simulink model "B2B_HVDC_MMC"  (R2023b)
settings: Solver=ode23t  StartTime=0.0  StopTime=3  FixedStep=Ts_Power  MaxStep=1e-3  MinStep=Ts_Power  RelTol=1e-3
values from neighbouring files (symbols this model uses):
  AC_lim = 1*[1.5 -1.5]    [B2B_HVDC_MMC_Calc.m]
  C_pm = 10.48e-3    (= 0.01048)    [B2B_HVDC_MMC_Calc.m]
  Carm = 1.0*C_pm/n    (= 0.0002096)    [B2B_HVDC_MMC_Calc.m]    (also in HVDC_MMC_param.m = 4.88333333333e-05)
  ccsc_lim = 1*[1.0 -1.0]    [B2B_HVDC_MMC_Calc.m]
  DC_lim = 1*[1.05 -1.05]    [B2B_HVDC_MMC_Calc.m]
  f = 50    [B2B_HVDC_MMC_Calc.m]
  Fn_filter = 1000    [B2B_HVDC_MMC_Calc.m]    (also in HVDC_MMC_param.m)
  Fnom = 50    [HVDC_MMC_param.m]
  HrmOrd = N    (= 2)    [B2B_HVDC_MMC_Calc.m]    (also in HVDC_MMC_param.m)
  I_nom = S_nom/(sqrt(3)*V_grid)    [B2B_HVDC_MMC_Calc.m]
  Ireg_lim_i = 1*[1.5, -1.5]    [B2B_HVDC_MMC_Calc.m]
  Ireg_lim_r = 2*[1.5, -1.5]    [B2B_HVDC_MMC_Calc.m]
  Ki_ACreg_i = 260    [B2B_HVDC_MMC_Calc.m]
  Ki_ccsc = 5    [B2B_HVDC_MMC_Calc.m]
  Ki_DCreg_r = 150    [B2B_HVDC_MMC_Calc.m]
  Ki_Ireg_i = 200    [B2B_HVDC_MMC_Calc.m]
  Ki_Ireg_r = 50    [B2B_HVDC_MMC_Calc.m]
  Kp_ACreg_i = 2    [B2B_HVDC_MMC_Calc.m]
  Kp_ccsc = 1    [B2B_HVDC_MMC_Calc.m]
  Kp_DCreg_r = 8    [B2B_HVDC_MMC_Calc.m]
  Kp_Ireg_i = 2    [B2B_HVDC_MMC_Calc.m]
  Kp_Ireg_r = 0.8    [B2B_HVDC_MMC_Calc.m]
  L1_si = L1_pu*Z_base66/w    [B2B_HVDC_MMC_Calc.m]
  L_arm = L_arm_pu*Z_base66/w    [B2B_HVDC_MMC_Calc.m]
  L_arm_pu = 0.15    [B2B_HVDC_MMC_Calc.m]
  N = 2    [B2B_HVDC_MMC_Calc.m]
  P_nom = 220e6    (= 220000000)    [B2B_HVDC_MMC_Calc.m]
  R1_si = R1_pu*Z_base66    [B2B_HVDC_MMC_Calc.m]
  R_arm = 0.03    [B2B_HVDC_MMC_Calc.m]
  R_arm_pu = R_arm/Z_base66    [B2B_HVDC_MMC_Calc.m]
  R_load = 0.6*40    (= 24)    [B2B_HVDC_MMC_Calc.m]
  R_startup = 17    [B2B_HVDC_MMC_Calc.m]    (also in HVDC_MMC_param.m = 400)
  T_fault = 1.4    [B2B_HVDC_MMC_Calc.m]
  Ts = Ts_Power    (= 5e-05)    [B2B_HVDC_MMC_Calc.m]    (also in HVDC_MMC_param.m)
  Ts_Control = Ts_Power    (= 5e-05)    [B2B_HVDC_MMC_Calc.m]    (also in HVDC_MMC_param.m)
  Ts_DQN = MultTs*Ts_Power    (= 5e-05)    [B2B_HVDC_MMC_Calc.m]    (also in HVDC_MMC_param.m)
  Ts_Power = 1*50e-6    (= 5e-05)    [B2B_HVDC_MMC_Calc.m]    (also in HVDC_MMC_param.m)
  V_ac_ref = 1.035    [B2B_HVDC_MMC_Calc.m]
  V_grid = 66e3    (= 66000)    [B2B_HVDC_MMC_Calc.m]
  Vdc_nom = 135e3    (= 135000)    [B2B_HVDC_MMC_Calc.m]
  Vnom_prim = 333e3    (= 333000)    [HVDC_MMC_param.m]
  Xdcpnz = [zeros(6,1), Xpnz]    [B2B_HVDC_MMC_Calc.m]
  Zeta_filter = 1    [B2B_HVDC_MMC_Calc.m]    (also in HVDC_MMC_param.m)
undefined symbols (not defined in the file or in its folder): DiscIntNeverNeededParam, Pcc, Xdcpnz_c
libraries: DQN_Lib x39, simulink x26, eeTransforms x21, spsCurrentMeasurementLib x16, spsHalfBridgeMMCLib x12, spsSeriesRLCBranchLib x12, B2B_HVDC_MMC_Lib x8, spsSecondOrderFilterLib x8, spsAlphaBetaZerotodq0Lib x6, spsabctoAlphaBetaZeroLib x6, spsThreePhaseVIMeasurementLib x4, spsabctodq0Lib x3
(part 2 of 5)

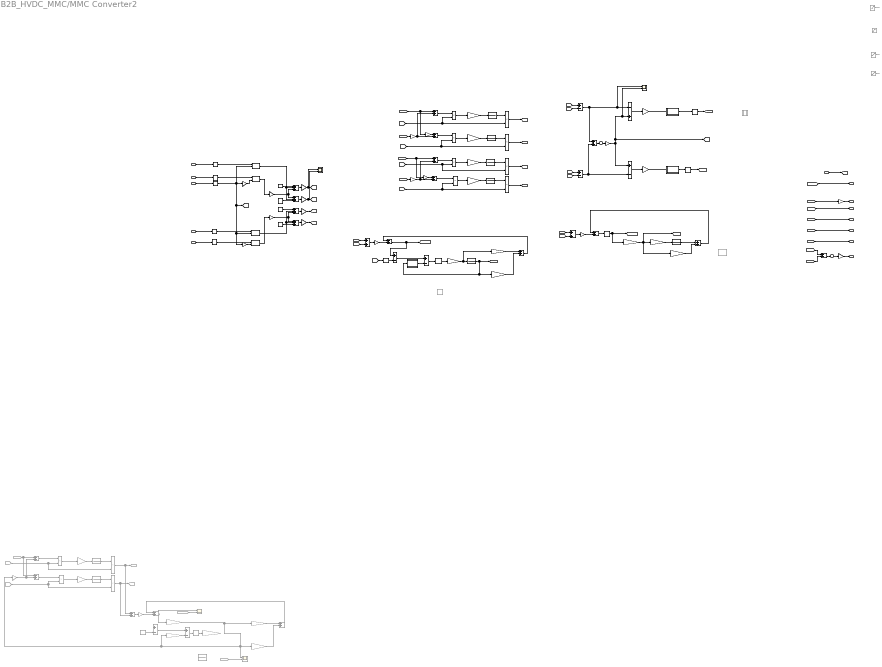
== system B2B_HVDC_MMC/MMC Converter2 ==
  m_dq1_r : Inport
  m_dq2_r : Inport  Port=2
  Vg : Inport  Port=3
  wt : Inport  Port=4
  m_dq1_i : Inport  Port=5
  m_dq2_i : Inport  Port=6
  Add1 : Sum  Inputs=+-
  Add{3,6,38..39,41,44,48,50,73} (9 alike) : Sum
  Add35 : Sum  Commented=on
  Add36 : Sum  Commented=on
  Add37 : Sum  Commented=on  Inputs=-+
  Add4 : Sum  Commented=on
  Add42 : Sum  Inputs=-+
  Add45 : Sum  Inputs=-+
  Add46 : Sum  Inputs=+-
  Add47 : Sum  Inputs=+-
  Add5 : Sum  Commented=on  Inputs=-+
  Constant : Constant  Commented=on  Value=0
  Constant{1..2,74..75} (4 alike) : Constant
  Delay : Delay  Commented=on  DelayLength=1  SampleTime=Ts_Power
  Delay{2..3,8..9} (4 alike) : Delay  DelayLength=1  SampleTime=Ts_Power
  Delay4 : Delay  Commented=on  DelayLength=1  SampleTime=Ts_Power
  Discrete Derivative : simulink/Discrete/Discrete Derivative  Commented=on  gainval=Ts_Power  ICPrevScaledInput=0.0  OutMin=[]  OutMax=[]  OutDataType=fixdt(1, 16)  OutScaling=2^-10  DoSatur=off
  Discrete-Time Integrator{,2..3,7,10..11} (6 alike) : DiscreteIntegrator  IntegratorMethod=Integration: Trapezoidal  SampleTime=Ts_Power  ICPrevOutput=DiscIntNeverNeededParam  ICPrevScaledInput=DiscIntNeverNeededParam
  Discrete-Time Integrator4 : DiscreteIntegrator  Commented=on  IntegratorMethod=Integration: Trapezoidal  SampleTime=Ts_Power  ICPrevOutput=DiscIntNeverNeededParam  ICPrevScaledInput=DiscIntNeverNeededParam
  Discrete-Time Integrator5 : DiscreteIntegrator  Commented=on  IntegratorMethod=Integration: Trapezoidal  SampleTime=Ts_Power  ICPrevOutput=DiscIntNeverNeededParam  ICPrevScaledInput=DiscIntNeverNeededParam
  Discrete-Time Integrator8 : DiscreteIntegrator  Commented=on  IntegratorMethod=Integration: Trapezoidal  SampleTime=Ts_Power  ICPrevOutput=DiscIntNeverNeededParam  ICPrevScaledInput=DiscIntNeverNeededParam
  From108 : From  Commented=on  GotoTag=Id_abc_i
  From51 : From  Commented=on  GotoTag=mn_i
  From56 : From  Commented=on  GotoTag=mp_i
  From72 : From  Commented=on  GotoTag=Ig_abc_i
  From75 : From  Commented=on  GotoTag=Vconv_i
  Gain{1..2,18,23..24} (5 alike) : Gain  Gain=-1
  Gain10 : Gain  Gain=1/6
  Gain12 : Gain  Gain=-2
  Gain13 : Gain  Commented=on  Gain=1/(Carm)
  Gain14 : Gain  Commented=on  Gain=1/(Carm)
  Gain15 : Gain  Commented=on  Gain=0.5
  Gain{4,21,39,43} (4 alike) : Gain  Gain=1/(Carm)
  Gain40 : Gain  Commented=on  Gain=-0.5
  Gain41 : Gain  Gain=1/2
  Gain44 : Gain  Gain=0.5
  Gain46 : Gain  Commented=on  Gain=1/R_load
  Gain47 : Gain  Gain=0.5
  Gain49 : Gain  Gain=-0.5
  Gain50 : Gain  Gain=1/R_load
  Gain51 : Gain  Gain=R_arm/2
  Gain52 : Gain  Commented=on  Gain=R_arm/2
  Gain53 : Gain  Commented=on  Gain=L_arm/2
  Gain54 : Gain  Commented=on  Gain=1/L1_si
  Gain55 : Gain  Commented=on  Gain=R1_si+R_load
  Gain56 : Gain  Gain=L_arm/2
  Gain60 : Gain  Gain=-0.5
  Gain61 : Gain  Gain=R_arm/2
  Gain62 : Gain  Gain=L_arm/2
  Gain65 : Gain  Gain=1/L1_si
  Gain9 : Gain  Gain=-2
  Goto56 : Goto  Commented=on  GotoTag=Vp_ic
  Goto57 : Goto  Commented=on  GotoTag=Vn_ic
  I->pu{1..3,5,22,28} (6 alike) : Gain  Gain=1/2  SaturateOnIntegerOverflow=on  OutDataTypeStr=Inherit: Same as input  ParamDataTypeStr=Inherit: Same as input
  Int : MATLAB Function  TreatAsAtomicUnit=on  mask{dt=Ts_Power}
      mask prompts: dt "Time step (s):"
  Int2 : MATLAB Function  TreatAsAtomicUnit=on  mask{dt=Ts_Power}
      mask prompts: dt "Time step (s):"
  Inverse Park Transform{1..4} (4 alike) : eeTransforms/Inverse Park Transform  AxisAlignment=Q-axis  PowerInvariant=off
  Product{1..3,5} (4 alike) : Product  Commented=on
  Product{4,6..12} (8 alike) : Product
  R_rec1 : Subsystem
  Rate Transition{1..4,10..11} (6 alike) : RateTransition  Integrity=off  OutPortSampleTimeMultiple=MultTs  OutPortSampleTime=Ts_Power
  Saturation3 : Saturate  Commented=on  UpperLimit=inf  LowerLimit=0  ZeroCross=off
  Saturation4 : Saturate  Commented=on  UpperLimit=inf  LowerLimit=0  ZeroCross=off
  Saturation5 : Saturate  Commented=on  UpperLimit=0  LowerLimit=-inf  ZeroCross=off
  Saturation6 : Saturate  Commented=on  UpperLimit=0  LowerLimit=-inf  ZeroCross=off
  Scope : Scope  NumInputPorts=2
  Scope1 : Scope  NumInputPorts=2
  Scope15 : Scope  Commented=on  NumInputPorts=2
  Scope8 : Scope  Commented=on  NumInputPorts=2
  Subsystem2 : Subsystem  Commented=on  mask{Ts_Power=Ts_Power, SW=off}
      mask prompts: Ts_Power "Sample time (s):"; SW "Fancy delay"
  Subtract1 : Sum  Inputs=+-+
  Subtract10 : Sum  Inputs=+-
  Subtract11 : Sum  Inputs=+-
  Subtract2 : Sum  Inputs=+-+
  Subtract3 : Sum  Inputs=+++
  Subtract4 : Sum  Commented=on  Inputs=+-
  Subtract5 : Sum  Inputs=+++
  Subtract8 : Sum  Commented=on  Inputs=+-
  Sum11 : Sum  Inputs=+-  InputSameDT=on  SaturateOnIntegerOverflow=on  OutDataTypeStr=Inherit: Same as first input
  Sum19 : Sum  Inputs=+
  Sum23 : Sum  Inputs=+
  Sum4 : Sum  Inputs=-+  InputSameDT=on  SaturateOnIntegerOverflow=on  OutDataTypeStr=Inherit: Same as first input
  Id_abc_i : Outport  VectorParamsAs1DForOutWhenUnconnected=off
  Ig_abc_i : Outport  Port=2  VectorParamsAs1DForOutWhenUnconnected=off
  Vg_abc_i : Outport  Port=3  VectorParamsAs1DForOutWhenUnconnected=off
  Idc : Outport  Port=4  VectorParamsAs1DForOutWhenUnconnected=off
  Ig_abc_r : Outport  Port=5  VectorParamsAs1DForOutWhenUnconnected=off
  Id_abc_r : Outport  Port=6  VectorParamsAs1DForOutWhenUnconnected=off
  Vdc : Outport  Port=7  VectorParamsAs1DForOutWhenUnconnected=off
  wires:
  Gain9/1 -> Inverse Park Transform2/2
  [mn_r] -> Product7/2, Product8/2
  Gain4/1 -> Discrete-Time Integrator3/1  "dVp_M"
  Gain21/1 -> Discrete-Time Integrator2/1  "dVn_M"
  Discrete-Time Integrator2/1 -> Product8/1  "Vn_M"
  Product4/1 -> Gain4/1
  Add6/1 -> Product7/1
  Add46/1 -> Scope1/1, Sum4/1, Add73/1  "dVp_M"
  Discrete-Time Integrator3/1 -> Product6/1  "Vp_M"
  Product7/1 -> Gain21/1
  Subtract2/1 -> I->pu22/1
  Constant74/1 -> Subtract2/1
  Inverse Park Transform2/1 -> Gain1/1
  Constant75/1 -> Subtract5/3
  Subtract5/1 -> I->pu28/1
  I->pu28/1 -> Scope/2, [mn_r]
  Inverse Park Transform1/1 -> Subtract5/2, Subtract2/2
  Gain12/1 -> Inverse Park Transform4/2
  wt/1 -> Rate Transition1/1
  Constant2/1 -> Subtract3/3
  Subtract1/1 -> I->pu2/1
  Constant1/1 -> Subtract1/1
  Subtract3/1 -> I->pu3/1
  I->pu2/1 -> [mp_i]
  Inverse Park Transform4/1 -> Gain2/1
  I->pu3/1 -> [mn_i]
  Gain15/1 -> Add4/2, Add5/2
  Discrete-Time Integrator5/1 -> Product2/1  "Vp_M"
  Add5/1 -> Product3/1
  Add4/1 -> Product1/1  "prod"
  Gain14/1 -> Discrete-Time Integrator5/1  "dVp_M"
  Product1/1 -> Gain14/1
  Discrete-Time Integrator4/1 -> Product5/1  "Vn_M"
  Gain13/1 -> Discrete-Time Integrator4/1  "dVn_M"
  Product3/1 -> Gain13/1
  From51/1 -> Product2/2, Product1/2
  From56/1 -> Product3/2, Product5/2
  Vg/1 -> [Vg_r]
  Sum4/1 -> I->pu5/1
  Gain23/1 -> Ig_abc_r/1
  Gain44/1 -> Add6/2, Add3/2
  From75/1 -> Scope8/2
  Constant/1 -> Subtract4/2
  Delay4/1 -> Gain54/1
  Gain55/1 -> Subtract8/2
  Subtract8/1 -> Delay4/1
  Gain53/1 -> Add36/1  "dVp_M"
  Gain52/1 -> Add36/2  "dVp_M"
  Add37/1 -> Scope8/1, Gain46/1  "prod"
  Subtract4/1 -> Subtract8/1
  Product2/1 -> Add35/1, Goto56/1
  Gain46/1 -> Scope15/1, Gain55/1, Gain15/1, Gain52/1, Gain53/1  "Igd"
  Product5/1 -> Add35/2, Goto57/1
  From72/1 -> Scope15/2
  Add36/1 -> Add37/1  "prod"
  Add35/1 -> Gain40/1
  Gain40/1 -> Add37/2  "Vce_i"
  From108/1 -> Add5/1, Add4/1
  Gain47/1 -> Add38/2, Add39/2
  Product11/1 -> Gain39/1
  [mp_i] -> Product11/2, Product12/2
  Add38/1 -> Product9/1  "prod"
  Discrete-Time Integrator11/1 -> Product10/1  "Vp_M"
  Gain39/1 -> Discrete-Time Integrator10/1  "dVn_M"
  Discrete-Time Integrator10/1 -> Product12/1  "Vn_M"
  Product9/1 -> Gain43/1
  Gain43/1 -> Discrete-Time Integrator11/1  "dVp_M"
  Add39/1 -> Product11/1
  [mn_i] -> Product10/2, Product9/2
  Add41/1 -> Add42/1  "prod"
  Gain51/1 -> Add41/2  "dVp_M"
  Add50/1 -> Gain49/1
  Gain49/1 -> Add42/2  "Vce_i"
  Subtract10/1 -> Subtract11/1
  Gain61/1 -> Add44/2  "dVp_M"
  Add44/1 -> Add45/1  "prod"
  Gain60/1 -> Add45/2  "Vce_r"
  Gain62/1 -> Add44/1  "dVp_M"
  R_rec1/1(Out) -> Subtract11/2
  Gain65/1 -> Discrete-Time Integrator/1, Gain62/1
  Add48/1 -> Gain60/1
  [Ig_abc_ic] -> Gain47/1
  [Id_abc_ic] -> Gain24/1, Add38/1
  [Vp_rc] -> Add46/1
  [Vn_rc] -> Add46/2
  [Vp_ic] -> Add47/1
  [Vn_ic] -> Add47/2
  [Ig_abc_rc] -> Gain44/1
  [Id_abc_rc] -> Add3/1, Gain18/1
  [Vp_rc] -> Add48/1
  [Vn_rc] -> Add48/2
  [Vp_ic] -> Add50/1
  [Vn_ic] -> Add50/2
  Add47/1 -> Sum11/2, Add73/2  "dVp_M"
  [Ig_abc_rc] -> Gain23/1
  [Id_abc_rc] -> Id_abc_r/1
  [Ig_abc_ic] -> Ig_abc_i/1
  [Id_abc_ic] -> Id_abc_i/1
  [Id_abc_rc] -> Add1/2
  Gain56/1 -> Discrete-Time Integrator7/1  "dVp_M"
  Discrete-Time Integrator7/1 -> Add41/1
  [Id_abc_ic] -> Add1/1
  Add1/1 -> Sum23/1
  Gain41/1 -> Idc/1  "Vce_r"
  Discrete-Time Integrator/1 -> [Ig_abc_rc], R_rec1/1(In), Gain61/1  "Igd"
  Add45/1 -> [Vconv_rc], Subtract10/1  "prod"
  Gain50/1 -> Gain51/1, [Ig_abc_ic], Gain56/1  "Igd"
  Add42/1 -> Delay8/1  "prod"
  [Vconv_ic] -> Vg_abc_i/1
  [V_dc_c] -> Vdc/1
  Subtract11/1 -> Delay9/1
  Gain1/1 -> Subtract5/1, Subtract2/3
  Inverse Park Transform3/1 -> Subtract1/2, Subtract3/2
  Gain2/1 -> Subtract3/1, Subtract1/3
  Gain10/1 -> Sum11/1, [V_dc_c], Scope1/2, Sum4/2  "Vce_r"
  m_dq2_r/1 -> Rate Transition11/1
  m_dq1_r/1 -> Rate Transition10/1
  m_dq1_i/1 -> Rate Transition2/1
  m_dq2_i/1 -> Rate Transition3/1
  Gain18/1 -> Add6/1
  Gain24/1 -> Add39/1
  Saturation4/1 -> ?
  Saturation3/1 -> ?
  Saturation6/1 -> ?
  Add73/1 -> Sum19/1
  Sum19/1 -> Gain10/1
  Int/1(z) -> Delay2/1
  Sum11/1 -> I->pu1/1
  Int2/1(z) -> Delay3/1
  Product6/1 -> [Vp_rc]
  Product8/1 -> [Vn_rc]
  Product10/1 -> [Vp_ic]
  Product12/1 -> [Vn_ic]
  Delay2/1 -> [Id_abc_rc]
  Delay3/1 -> [Id_abc_ic]
  Delay9/1 -> Gain65/1
  Delay8/1 -> Gain50/1, [Vconv_ic]
  I->pu5/1 -> Int/1(x)
  I->pu1/1 -> Int2/1(x)
  Rate Transition10/1 -> Inverse Park Transform1/1
  Rate Transition11/1 -> Inverse Park Transform2/1
  Rate Transition1/1 -> [wt], Inverse Park Transform3/2, Gain12/1, Inverse Park Transform1/2, Gain9/1
  Rate Transition2/1 -> Inverse Park Transform3/1
  Rate Transition3/1 -> Inverse Park Transform4/1
  [Vg_r] -> Rate Transition4/1
  Rate Transition4/1 -> Subtract10/2
  Sum23/1 -> Gain41/1
  I->pu22/1 -> Scope/1, [mp_r]
  Add3/1 -> Product4/1  "prod"
  [mp_r] -> Product4/2, Product6/2

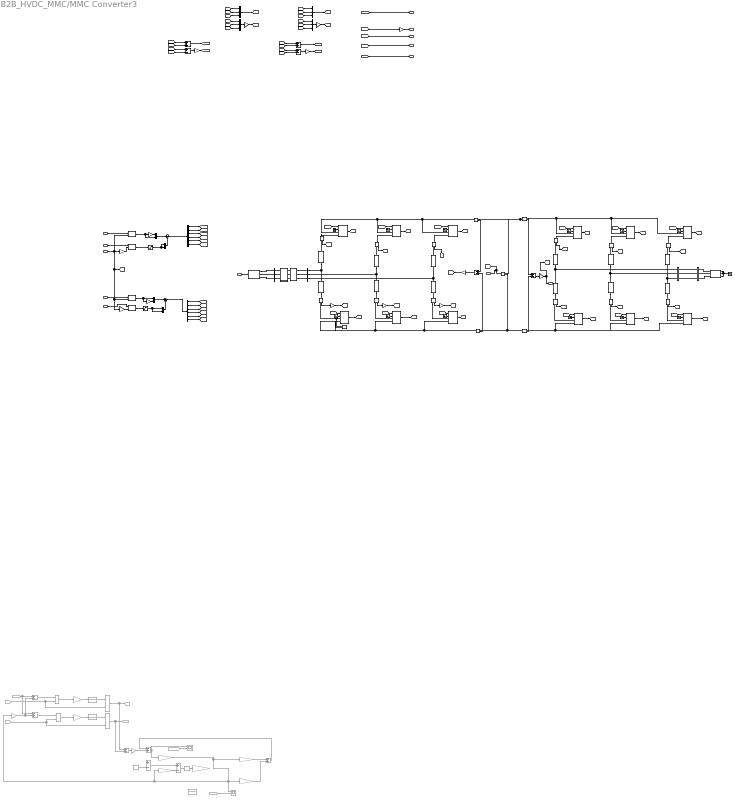
== system B2B_HVDC_MMC/MMC Converter3 ==
  m_dq1_r : Inport
  m_dq2_r : Inport  Port=2
  wt : Inport  Port=3
  V_Src : Inport  Port=4
  m_dq1_i : Inport  Port=5
  m_dq2_i : Inport  Port=6
  A1 : spsThreePhaseVIMeasurementLib/Three-Phase V-I Measurement  VoltageMeasurement=phase-to-ground  SetLabelV=on  LabelV=Vconv_r  Vpu=off  VpuLL=off  CurrentMeasurement=yes  SetLabelI=on  LabelI=Ig_r  Ipu=off  Pbase=100e6  Vbase=500e3  OutputType=Complex  PhasorSimulation=off  PSBequivalent=0
  A2 : spsThreePhaseVIMeasurementLib/Three-Phase V-I Measurement  VoltageMeasurement=phase-to-ground  SetLabelV=on  LabelV=Vconv_i  Vpu=off  VpuLL=off  CurrentMeasurement=yes  SetLabelI=on  LabelI=Ig_i  Ipu=off  Pbase=100e6  Vbase=500e3  OutputType=Complex  PhasorSimulation=off  PSBequivalent=0
  A3 : spsThreePhaseVIMeasurementLib/Three-Phase V-I Measurement  VoltageMeasurement=phase-to-ground  SetLabelV=on  LabelV=VA1  Vpu=off  VpuLL=off  CurrentMeasurement=yes  SetLabelI=on  LabelI=IA1  Ipu=off  Pbase=100e6  Vbase=500e3  OutputType=Complex  PhasorSimulation=off  PSBequivalent=0
  Add : Sum
  Add{8,11,13,51} (4 alike) : Sum  Inputs=+-
  Add35 : Sum  Commented=on
  Add36 : Sum  Commented=on
  Add37 : Sum  Commented=on  Inputs=-+
  Add4 : Sum  Commented=on
  Add40 : Sum
  Add5 : Sum  Commented=on  Inputs=-+
  B1 : spsThreePhaseVIMeasurementLib/Three-Phase V-I Measurement  VoltageMeasurement=phase-to-ground  SetLabelV=on  LabelV=VB1  Vpu=off  VpuLL=off  CurrentMeasurement=yes  SetLabelI=on  LabelI=IB1  Ipu=off  Pbase=100e6  Vbase=500e3  OutputType=Complex  PhasorSimulation=off  PSBequivalent=0
  Constant : Constant  Commented=on  Value=0
  Current Measurement{,1..15} (16 alike) : spsCurrentMeasurementLib/Current Measurement  PhasorSimulation=off  OutputType=Complex  PSBequivalent=0
  Delay4 : Delay  Commented=on  DelayLength=1  SampleTime=Ts_Power
  Demux1 : Demux  Outputs=6
  Demux2 : Demux  Outputs=6
  Discrete-Time Integrator4 : DiscreteIntegrator  Commented=on  IntegratorMethod=Integration: Trapezoidal  SampleTime=Ts_Power  ICPrevOutput=DiscIntNeverNeededParam  ICPrevScaledInput=DiscIntNeverNeededParam
  Discrete-Time Integrator5 : DiscreteIntegrator  Commented=on  IntegratorMethod=Integration: Trapezoidal  SampleTime=Ts_Power  ICPrevOutput=DiscIntNeverNeededParam  ICPrevScaledInput=DiscIntNeverNeededParam
  Discrete-Time Integrator8 : DiscreteIntegrator  Commented=on  IntegratorMethod=Integration: Trapezoidal  SampleTime=Ts_Power  ICPrevOutput=DiscIntNeverNeededParam  ICPrevScaledInput=DiscIntNeverNeededParam
  From108 : From  Commented=on  GotoTag=Id_abc_i
  From51 : From  Commented=on  GotoTag=mn_i
  From56 : From  Commented=on  GotoTag=mp_i
  From72 : From  Commented=on  GotoTag=Ig_abc_i
  From75 : From  Commented=on  GotoTag=Vconv_i
  Gain{,24,34,37} (4 alike) : Gain  Gain=0.5
  Gain{2,5,11,18,23} (5 alike) : Gain  Gain=-1
  Gain12 : Gain  Gain=-2
  Gain13 : Gain  Commented=on  Gain=1/(Carm)
  Gain14 : Gain  Commented=on  Gain=1/(Carm)
  Gain15 : Gain  Commented=on  Gain=0.5
  Gain19 : Gain
  Gain20 : Gain
  Gain22 : Gain
  Gain40 : Gain  Commented=on  Gain=-0.5
  Gain46 : Gain  Commented=on  Gain=1/R_load
  Gain52 : Gain  Commented=on  Gain=R_arm/2
  Gain53 : Gain  Commented=on  Gain=L_arm/2
  Gain54 : Gain  Commented=on  Gain=1/L1_si
  Gain55 : Gain  Commented=on  Gain=R1_si+R_load
  Gain9 : Gain  Gain=-2
  Goto56 : Goto  Commented=on  GotoTag=Vp_ic
  Goto57 : Goto  Commented=on  GotoTag=Vn_ic
  Ground{,1..11} (12 alike) : Ground
  Ground12 : spsGroundLib/Ground  LConnTagsString=a
  Half-Bridge MMC{,1..11} (12 alike) : spsHalfBridgeMMCLib/Half-Bridge MMC  ModelType=Average model (Uref-controlled)  n=n  C=C_pm  Vc_Initial=Vc_pm_r  Ron=1e-3  Rs=1e6  Cs=inf  Ron_Diode=1e-6  Rs_Diode=1e9  Cs_Diode=inf  Vf_Diode=0  Rs_CurrentSource=inf  Ts=Ts_Power
  Inverse Park Transform{1..4} (4 alike) : eeTransforms/Inverse Park Transform  AxisAlignment=Q-axis  PowerInvariant=off
  Mux{1,4,32..33} (4 alike) : Mux  Inputs=3
  Mux{6..7,15..16} (4 alike) : Mux  Inputs=2
  Product{1..3,5} (4 alike) : Product  Commented=on
  R_startup1 : spsThreePhaseSeriesRLCBranchLib/Three-Phase Series RLC Branch  LConnTagsString=A|B|C  RConnTagsString=A|B|C  BranchType=RL  Resistance=R1_si  Inductance=L1_si  Capacitance=1e-6  Measurements=None
  Saturation1 : Saturate  UpperLimit=ccsc_lim(1)  LowerLimit=ccsc_lim(2)
  Saturation2 : Saturate  UpperLimit=ccsc_lim(1)  LowerLimit=ccsc_lim(2)
  Scope15 : Scope  Commented=on  NumInputPorts=2
  Scope8 : Scope  Commented=on  NumInputPorts=2
  Subsystem5 : Subsystem
      mask Display:
      | color('blue')
      | disp('Startup')
  Subtract4 : Sum  Commented=on  Inputs=+-
  Subtract8 : Sum  Commented=on  Inputs=+-
  Sum : Sum  Inputs=|+-
  Sum10 : Sum  Inputs=|+-
  Three-Phase Series RLC Branch : spsThreePhaseSeriesRLCBranchLib/Three-Phase Series RLC Branch  LConnTagsString=A|B|C  RConnTagsString=A|B|C  BranchType=R  Resistance=R_load  Inductance=1e-3  Capacitance=1e-6  Measurements=None
  Unai : spsSeriesRLCBranchLib/Series RLC Branch  LConnTagsString=__new0  RConnTagsString=__new0  BranchType=RL  Resistance=R_arm  Inductance=L_arm  SetiL0=off  InitialCurrent=0  Capacitance=1e-6  Setx0=off  InitialVoltage=0  Measurements=Branch voltage
  Unar : spsSeriesRLCBranchLib/Series RLC Branch  LConnTagsString=__new0  RConnTagsString=__new0  BranchType=RL  Resistance=R_arm  Inductance=L_arm  SetiL0=off  InitialCurrent=0  Capacitance=1e-6  Setx0=off  InitialVoltage=0  Measurements=Branch voltage
  Unbi : spsSeriesRLCBranchLib/Series RLC Branch  LConnTagsString=__new0  RConnTagsString=__new0  BranchType=RL  Resistance=R_arm  Inductance=L_arm  SetiL0=off  InitialCurrent=0  Capacitance=1e-6  Setx0=off  InitialVoltage=0  Measurements=Branch voltage
  Unbr : spsSeriesRLCBranchLib/Series RLC Branch  LConnTagsString=__new0  RConnTagsString=__new0  BranchType=RL  Resistance=R_arm  Inductance=L_arm  SetiL0=off  InitialCurrent=0  Capacitance=1e-6  Setx0=off  InitialVoltage=0  Measurements=Branch voltage
  Unci : spsSeriesRLCBranchLib/Series RLC Branch  LConnTagsString=__new0  RConnTagsString=__new0  BranchType=RL  Resistance=R_arm  Inductance=L_arm  SetiL0=off  InitialCurrent=0  Capacitance=1e-6  Setx0=off  InitialVoltage=0  Measurements=Branch voltage
  Uncr : spsSeriesRLCBranchLib/Series RLC Branch  LConnTagsString=__new0  RConnTagsString=__new0  BranchType=RL  Resistance=R_arm  Inductance=L_arm  SetiL0=off  InitialCurrent=0  Capacitance=1e-6  Setx0=off  InitialVoltage=0  Measurements=Branch voltage
  Upai : spsSeriesRLCBranchLib/Series RLC Branch  LConnTagsString=__new0  RConnTagsString=__new0  BranchType=RL  Resistance=R_arm  Inductance=L_arm  SetiL0=off  InitialCurrent=0  Capacitance=1e-6  Setx0=off  InitialVoltage=0  Measurements=Branch voltage
  Upar : spsSeriesRLCBranchLib/Series RLC Branch  LConnTagsString=__new0  RConnTagsString=__new0  BranchType=RL  Resistance=R_arm  Inductance=L_arm  SetiL0=off  InitialCurrent=0  Capacitance=1e-6  Setx0=off  InitialVoltage=0  Measurements=Branch voltage
  Upbi : spsSeriesRLCBranchLib/Series RLC Branch  LConnTagsString=__new0  RConnTagsString=__new0  BranchType=RL  Resistance=R_arm  Inductance=L_arm  SetiL0=off  InitialCurrent=0  Capacitance=1e-6  Setx0=off  InitialVoltage=0  Measurements=Branch voltage
  Upbr : spsSeriesRLCBranchLib/Series RLC Branch  LConnTagsString=__new0  RConnTagsString=__new0  BranchType=RL  Resistance=R_arm  Inductance=L_arm  SetiL0=off  InitialCurrent=0  Capacitance=1e-6  Setx0=off  InitialVoltage=0  Measurements=Branch voltage
  Upci : spsSeriesRLCBranchLib/Series RLC Branch  LConnTagsString=__new0  RConnTagsString=__new0  BranchType=RL  Resistance=R_arm  Inductance=L_arm  SetiL0=off  InitialCurrent=0  Capacitance=1e-6  Setx0=off  InitialVoltage=0  Measurements=Branch voltage
  Upcr : spsSeriesRLCBranchLib/Series RLC Branch  LConnTagsString=__new0  RConnTagsString=__new0  BranchType=RL  Resistance=R_arm  Inductance=L_arm  SetiL0=off  InitialCurrent=0  Capacitance=1e-6  Setx0=off  InitialVoltage=0  Measurements=Branch voltage
  Voltage Measurement : spsVoltageMeasurementLib/Voltage Measurement  PhasorSimulation=off  OutputType=Complex  PSBequivalent=0
  Voltage Measurement4 : spsVoltageMeasurementLib/Voltage Measurement  PhasorSimulation=off  OutputType=Complex  PSBequivalent=0
  Voltage source : Subsystem
  Id_abc_i : Outport  VectorParamsAs1DForOutWhenUnconnected=off
  Ig_abc_i : Outport  Port=2  VectorParamsAs1DForOutWhenUnconnected=off
  Vconv_i : Outport  Port=3  VectorParamsAs1DForOutWhenUnconnected=off
  I_dc : Outport  Port=4  VectorParamsAs1DForOutWhenUnconnected=off
  Ig_abc_r : Outport  Port=5  VectorParamsAs1DForOutWhenUnconnected=off
  Id_abc_r : Outport  Port=6  VectorParamsAs1DForOutWhenUnconnected=off
  V_dc : Outport  Port=7  VectorParamsAs1DForOutWhenUnconnected=off
  wires:
  Half-Bridge MMC3/1 -> [Vc2_r]
  Current Measurement2/1 -> [Ibu_r]
  Current Measurement3/1 -> [Icu_r]
  Current Measurement/1 -> [Iau_r]
  Half-Bridge MMC4/1 -> [Vc4_r]
  Half-Bridge MMC1/1 -> [Vc3_r]
  Demux1/1 -> [uref_apr]
  Demux1/5 -> [uref_bnr]
  Demux1/4 -> [uref_anr]
  Demux1/3 -> [uref_cpr]
  Demux1/6 -> [uref_cnr]
  Demux1/2 -> [uref_bpr]
  [uref_apr] -> Half-Bridge MMC/1
  Half-Bridge MMC/1 -> [Vc1_r]
  Ground/1 -> Half-Bridge MMC/2
  Ground1/1 -> Half-Bridge MMC1/2
  [uref_bpr] -> Half-Bridge MMC1/1
  Half-Bridge MMC2/1 -> [Vc5_r]
  Ground2/1 -> Half-Bridge MMC2/2
  [uref_cpr] -> Half-Bridge MMC2/1
  Ground3/1 -> Half-Bridge MMC3/2
  [uref_anr] -> Half-Bridge MMC3/1
  [uref_bnr] -> Half-Bridge MMC4/1
  Ground4/1 -> Half-Bridge MMC4/2
  Half-Bridge MMC5/1 -> [Vc6_r]
  [uref_cnr] -> Half-Bridge MMC5/1
  Ground5/1 -> Half-Bridge MMC5/2
  Ground11/1 -> Half-Bridge MMC11/2
  [uref_cni] -> Half-Bridge MMC11/1
  Current Measurement6/1 -> [Iau_i]
  Ground8/1 -> Half-Bridge MMC8/2
  Demux2/5 -> [uref_bni]
  Demux2/4 -> [uref_ani]
  Half-Bridge MMC11/1 -> [Vc6_i]
  [uref_bpi] -> Half-Bridge MMC7/1
  [uref_ani] -> Half-Bridge MMC9/1
  Demux2/6 -> [uref_cni]
  Ground9/1 -> Half-Bridge MMC9/2
  Half-Bridge MMC7/1 -> [Vc3_i]
  [uref_bni] -> Half-Bridge MMC10/1
  Demux2/3 -> [uref_cpi]
  Ground6/1 -> Half-Bridge MMC6/2
  Current Measurement11/1 -> [Icl_i]
  Demux2/2 -> [uref_bpi]
  [uref_api] -> Half-Bridge MMC6/1
  Half-Bridge MMC9/1 -> [Vc2_i]
  Current Measurement10/1 -> [Ibl_i]
  Half-Bridge MMC6/1 -> [Vc1_i]
  Ground10/1 -> Half-Bridge MMC10/2
  [uref_cpi] -> Half-Bridge MMC8/1
  Ground7/1 -> Half-Bridge MMC7/2
  Current Measurement7/1 -> [Ial_i]
  Half-Bridge MMC8/1 -> [Vc5_i]
  Half-Bridge MMC10/1 -> [Vc4_i]
  Current Measurement9/1 -> [Icu_i]
  Current Measurement8/1 -> [Ibu_i]
  Demux2/1 -> [uref_api]
  Voltage Measurement/1 -> V_dc/1, [V_dc]
  Saturation1/1 -> Mux6/1, Mux6/2
  m_dq1_r/1 -> Inverse Park Transform1/1
  Mux7/1 -> Sum/1
  Mux6/1 -> Sum/2
  Gain2/1 -> Mux7/1
  m_dq2_r/1 -> Inverse Park Transform2/1
  Gain9/1 -> Inverse Park Transform2/2
  Inverse Park Transform2/1 -> Saturation1/1
  Inverse Park Transform1/1 -> Mux7/2, Gain2/1
  Saturation2/1 -> Mux15/2, Mux15/1
  Mux16/1 -> Sum10/1
  Gain11/1 -> Mux16/2
  Mux15/1 -> Sum10/2
  Gain12/1 -> Inverse Park Transform4/2
  m_dq1_i/1 -> Inverse Park Transform3/1
  wt/1 -> [wt], Inverse Park Transform3/2, Gain12/1, Gain9/1, Inverse Park Transform1/2
  Sum10/1 -> Demux2/1
  m_dq2_i/1 -> Inverse Park Transform4/1
  Inverse Park Transform4/1 -> Saturation2/1
  Inverse Park Transform3/1 -> Gain11/1, Mux16/1
  Sum/1 -> Demux1/1
  Gain15/1 -> Add4/2, Add5/2
  Discrete-Time Integrator5/1 -> Product2/1  "Vp_M"
  Add5/1 -> Product3/1
  Add4/1 -> Product1/1  "prod"
  Gain14/1 -> Discrete-Time Integrator5/1  "dVp_M"
  Product1/1 -> Gain14/1
  Discrete-Time Integrator4/1 -> Product5/1  "Vn_M"
  Gain13/1 -> Discrete-Time Integrator4/1  "dVn_M"
  Product3/1 -> Gain13/1
  From51/1 -> Product2/2, Product1/2
  From56/1 -> Product3/2, Product5/2
  Current Measurement1/1 -> Gain19/1
  Gain19/1 -> [Ial_r]
  Current Measurement4/1 -> Gain20/1
  Gain20/1 -> [Ibl_r]
  Current Measurement5/1 -> Gain22/1
  Gain22/1 -> [Icl_r]
  Current Measurement12/1 -> Add8/1
  Current Measurement14/1 -> Add8/2
  Add8/1 -> Gain24/1
  Gain24/1 -> I_dc/1, [Idc_i]
  Gain23/1 -> Ig_abc_r/1
  From75/1 -> Scope8/2
  Constant/1 -> Subtract4/2
  Delay4/1 -> Gain54/1
  Gain55/1 -> Subtract8/2
  Subtract8/1 -> Delay4/1
  Gain53/1 -> Add36/1  "dVp_M"
  Gain52/1 -> Add36/2  "dVp_M"
  Add37/1 -> Scope8/1, Gain46/1  "prod"
  Subtract4/1 -> Subtract8/1
  Product2/1 -> Add35/1, Goto56/1
  Gain46/1 -> Scope15/1, Gain55/1, Gain15/1, Gain52/1, Gain53/1  "Igd"
  Product5/1 -> Add35/2, Goto57/1
  From72/1 -> Scope15/2
  Add36/1 -> Add37/1  "prod"
  Add35/1 -> Gain40/1
  Gain40/1 -> Add37/2  "Vce_i"
  Current Measurement13/1 -> Add13/1
  Current Measurement15/1 -> Add13/2
  Add13/1 -> Gain34/1
  Gain34/1 -> [Idc_r]
  From108/1 -> Add5/1, Add4/1
  [Icu_r] -> Mux32/3
  [Ibu_r] -> Mux32/2
  [Iau_r] -> Mux32/1
  [Ibl_r] -> Mux33/2
  [Ial_r] -> Mux33/1
  [Icl_r] -> Mux33/3
  Mux32/1 -> [Ip_r]
  Mux33/1 -> Gain5/1
  [Ip_r] -> Add/1
  [In_r] -> Add/2
  Gain5/1 -> [In_r]
  Add/1 -> [Ig_abc_r]
  [Ip_r] -> Add11/1
  [In_r] -> Add11/2
  Add11/1 -> Gain/1
  [Ig_abc_r] -> Gain23/1
  [Id_abc_r] -> Id_abc_r/1
  Gain/1 -> [Id_abc_r]
  [Icu_i] -> Mux1/3
  [Ial_i] -> Mux4/1
  Gain18/1 -> [In_i]
  Mux1/1 -> [Ip_i]
  [Ibu_i] -> Mux1/2
  [Iau_i] -> Mux1/1
  [Icl_i] -> Mux4/3
  [Ibl_i] -> Mux4/2
  Mux4/1 -> Gain18/1
  [Ip_i] -> Add40/1
  [In_i] -> Add40/2
  Add51/1 -> Gain37/1
  [Ip_i] -> Add51/1
  [In_i] -> Add51/2
  Add40/1 -> [Ig_abc_i]
  Gain37/1 -> [Id_abc_i]
  [Ig_abc_i] -> Ig_abc_i/1
  [Id_abc_i] -> Id_abc_i/1
  [Vconv_i] -> Vconv_i/1
  V_Src/1 -> Voltage source/1(In1)
  connections:
  Upbr/RConn1 -- A1/LConn2 -- Unbr/LConn1
  Unar/RConn1 -- Current Measurement1/LConn1
  Uncr/LConn1 -- A1/LConn3 -- Upcr/RConn1
  Upar/RConn1 -- A1/LConn1 -- Unar/LConn1
  Upbr/LConn1 -- Current Measurement2/RConn1
  Unbr/RConn1 -- Current Measurement4/LConn1
  Current Measurement5/LConn1 -- Uncr/RConn1
  Upcr/LConn1 -- Current Measurement3/RConn1
  Current Measurement/LConn1 -- Half-Bridge MMC/LConn2
  Upar/LConn1 -- Current Measurement/RConn1
  Half-Bridge MMC1/LConn2 -- Current Measurement2/LConn1
  Current Measurement3/LConn1 -- Half-Bridge MMC2/LConn2
  Half-Bridge MMC3/LConn1 -- Voltage Measurement4/LConn1 -- Current Measurement1/RConn1
  Half-Bridge MMC4/LConn1 -- Current Measurement4/RConn1
  Current Measurement5/RConn1 -- Half-Bridge MMC5/LConn1
  Unci/LConn1 -- A2/LConn3 -- Upci/RConn1
  Upbi/RConn1 -- A2/LConn2 -- Unbi/LConn1
  Half-Bridge MMC5/LConn2 -- Current Measurement15/LConn1 -- Half-Bridge MMC4/LConn2 -- Voltage Measurement4/LConn2 -- Half-Bridge MMC3/LConn2
  Half-Bridge MMC7/LConn1 -- Half-Bridge MMC8/LConn1 -- Half-Bridge MMC6/LConn1 -- Current Measurement12/RConn1
  Upai/RConn1 -- A2/LConn1 -- Unai/LConn1
  Half-Bridge MMC10/LConn1 -- Current Measurement10/RConn1
  Upai/LConn1 -- Current Measurement6/RConn1
  Half-Bridge MMC9/LConn1 -- Current Measurement7/RConn1
  Unbi/RConn1 -- Current Measurement10/LConn1
  Current Measurement11/LConn1 -- Unci/RConn1
  Current Measurement11/RConn1 -- Half-Bridge MMC11/LConn1
  Current Measurement9/LConn1 -- Half-Bridge MMC8/LConn2
  Half-Bridge MMC7/LConn2 -- Current Measurement8/LConn1
  Upci/LConn1 -- Current Measurement9/RConn1
  Upbi/LConn1 -- Current Measurement8/RConn1
  Current Measurement6/LConn1 -- Half-Bridge MMC6/LConn2
  Unai/RConn1 -- Current Measurement7/LConn1
  Current Measurement13/LConn1 -- Half-Bridge MMC2/LConn1 -- Half-Bridge MMC1/LConn1 -- Half-Bridge MMC/LConn1
  Half-Bridge MMC11/LConn2 -- Half-Bridge MMC10/LConn2 -- Half-Bridge MMC9/LConn2 -- Current Measurement14/RConn1
  Current Measurement12/LConn1 -- Current Measurement13/RConn1 -- Voltage Measurement/LConn1
  Current Measurement15/RConn1 -- Current Measurement14/LConn1 -- Voltage Measurement/LConn2
  R_startup1/RConn1 -- A1/RConn1
  R_startup1/RConn2 -- A1/RConn2
  R_startup1/RConn3 -- A1/RConn3
  B1/LConn3 -- A2/RConn3
  B1/LConn2 -- A2/RConn2
  B1/LConn1 -- A2/RConn1
  Voltage source/RConn1 -- A3/LConn1
  Voltage source/RConn2 -- A3/LConn2
  Voltage source/RConn3 -- A3/LConn3
  Subsystem5/LConn2 -- A3/RConn2
  R_startup1/LConn3 -- Subsystem5/RConn3
  Subsystem5/LConn1 -- A3/RConn1
  R_startup1/LConn2 -- Subsystem5/RConn2
  R_startup1/LConn1 -- Subsystem5/RConn1
  Subsystem5/LConn3 -- A3/RConn3
  Three-Phase Series RLC Branch/RConn1 -- Three-Phase Series RLC Branch/RConn2 -- Ground12/LConn1 -- Three-Phase Series RLC Branch/RConn3
  Three-Phase Series RLC Branch/LConn2 -- B1/RConn2
  Three-Phase Series RLC Branch/LConn1 -- B1/RConn1
  Three-Phase Series RLC Branch/LConn3 -- B1/RConn3

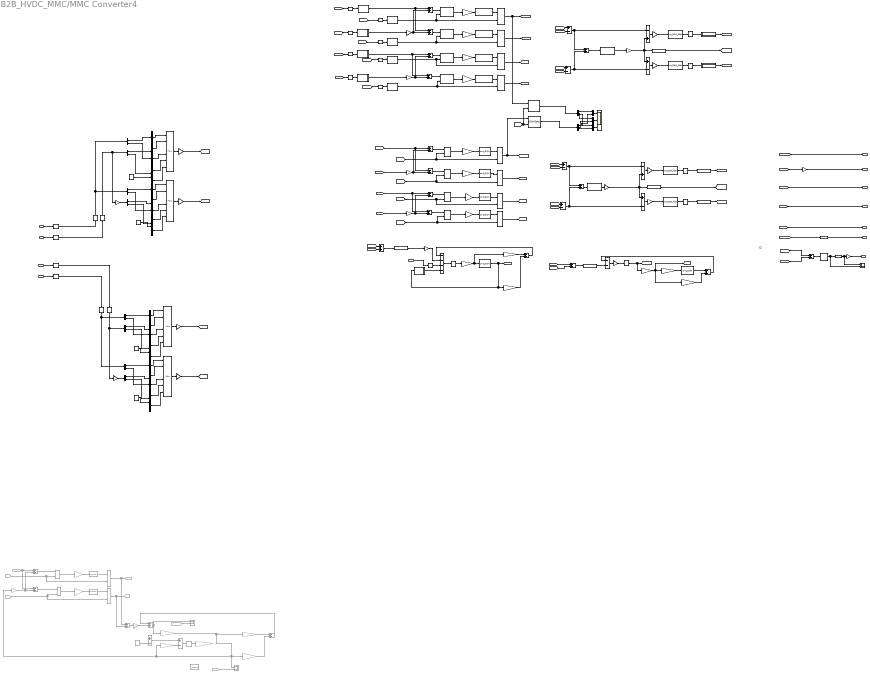
== system B2B_HVDC_MMC/MMC Converter4 ==
  m_dq1_r : Inport
  m_dq2_r : Inport  Port=2
  Vg_DQN : Inport  Port=3
  m_dq1_i : Inport  Port=4
  m_dq2_i : Inport  Port=5
  Add{,2..3,6,9..12,20..21} (10 alike) : Sum
  Add{1,14,17..19} (5 alike) : Sum  Inputs=+-
  Add13 : Sum  Inputs=--
  Add{7..8,15..16} (4 alike) : Sum  Inputs=-+
  Add35 : Sum  Commented=on
  Add36 : Sum  Commented=on
  Add37 : Sum  Commented=on  Inputs=-+
  Add4 : Sum  Commented=on
  Add5 : Sum  Commented=on  Inputs=-+
  Constant : Constant  Commented=on  Value=0
  Constant3 : Constant
  Constant4 : Constant  Value=-1
  Constant5 : Constant
  Constant6 : Constant  Value=-1
  DQn->ABC9 : DQN_Lib/DQn->ABC6  N=4*HrmOrd
  Delay{1..3,5,7..8} (6 alike) : Delay  DelayLength=1  SampleTime=Ts_Power
  Delay4 : Delay  Commented=on  DelayLength=1  SampleTime=Ts_Power
  Demux{,1..7} (8 alike) : Demux  Outputs=2
  Demux34 : Demux  Outputs=3
  Demux35 : Demux  Outputs=3
  Discrete-Time Integrator4 : DiscreteIntegrator  Commented=on  IntegratorMethod=Integration: Trapezoidal  SampleTime=Ts_Power  ICPrevOutput=DiscIntNeverNeededParam  ICPrevScaledInput=DiscIntNeverNeededParam
  Discrete-Time Integrator5 : DiscreteIntegrator  Commented=on  IntegratorMethod=Integration: Trapezoidal  SampleTime=Ts_Power  ICPrevOutput=DiscIntNeverNeededParam  ICPrevScaledInput=DiscIntNeverNeededParam
  Discrete-Time Integrator8 : DiscreteIntegrator  Commented=on  IntegratorMethod=Integration: Trapezoidal  SampleTime=Ts_Power  ICPrevOutput=DiscIntNeverNeededParam  ICPrevScaledInput=DiscIntNeverNeededParam
  From108 : From  Commented=on  GotoTag=Id_abc_i
  From51 : From  Commented=on  GotoTag=mn_i
  From56 : From  Commented=on  GotoTag=mp_i
  From72 : From  Commented=on  GotoTag=Ig_abc_i
  From75 : From  Commented=on  GotoTag=Vconv_i
  Gain1 : Gain  Gain=-1
  Gain10 : Gain  Gain=1/6
  Gain{8..9,11,22,36..37} (6 alike) : Gain  Gain=0.5
  Gain13 : Gain  Commented=on  Gain=1/(Carm)
  Gain14 : Gain  Commented=on  Gain=1/(Carm)
  Gain15 : Gain  Commented=on  Gain=0.5
  Gain16 : Gain  Gain=R_arm/2
  Gain19 : Gain  Gain=L_arm/2
  Gain{2,4..5,7,31,33..35} (8 alike) : Gain  Gain=1/(Carm)
  Gain20 : Gain  Gain=1/L1_si
  Gain25 : Gain  Gain=1/R_load
  Gain26 : Gain  Gain=R_arm
  Gain29 : Gain  Gain=L_arm
  Gain3 : Gain  Gain=-1
  Gain38 : Gain  Gain=1/6
  Gain40 : Gain  Commented=on  Gain=-0.5
  Gain41 : Gain  Gain=1/2
  Gain46 : Gain  Commented=on  Gain=1/R_load
  Gain52 : Gain  Commented=on  Gain=R_arm/2
  Gain53 : Gain  Commented=on  Gain=L_arm/2
  Gain54 : Gain  Commented=on  Gain=1/L1_si
  Gain55 : Gain  Commented=on  Gain=R1_si+R_load
  Gain6 : Gain  Gain=-1
  Goto56 : Goto  Commented=on  GotoTag=Vp_ic
  Goto57 : Goto  Commented=on  GotoTag=Vn_ic
  I->pu{1..3,9,12..13} (6 alike) : Gain  Gain=1/2  SaturateOnIntegerOverflow=on  OutDataTypeStr=Inherit: Same as input  ParamDataTypeStr=Inherit: Same as input
  I->pu10 : Gain  Gain=-1/2  SaturateOnIntegerOverflow=on  OutDataTypeStr=Inherit: Same as input  ParamDataTypeStr=Inherit: Same as input
  I->pu4 : Gain  Gain=-1/2  SaturateOnIntegerOverflow=on  OutDataTypeStr=Inherit: Same as input  ParamDataTypeStr=Inherit: Same as input
  Int_DQNc_Mat{1..4} (4 alike) : DQN_Lib/Int_DQNc_Mat  N=2*HrmOrd  dt=Ts_Power  w=w  InitInt=0*[0.8; 0.6; -0.33]  swFeed=off  R=1  iL=1
  MATLAB Function : MATLAB Function  TreatAsAtomicUnit=on
  MATLAB Function1 : MATLAB Function  TreatAsAtomicUnit=on
  MATLAB Function2 : MATLAB Function  TreatAsAtomicUnit=on
  MATLAB Function3 : MATLAB Function  TreatAsAtomicUnit=on
  MATLAB Function4 : MATLAB Function  TreatAsAtomicUnit=on
  MATLAB Function5 : MATLAB Function  TreatAsAtomicUnit=on
  MATLAB Function6 : MATLAB Function  TreatAsAtomicUnit=on
  MATLAB Function7 : MATLAB Function  TreatAsAtomicUnit=on
  Mult_DQNc_Mat{1..4} (4 alike) : DQN_Lib/Mult_DQNc_Mat  N=HrmOrd  HrmDbl=on
  Mult_DQNc_Mat{5..8} (4 alike) : DQN_Lib/Mult_DQNc_Mat  N=2*HrmOrd  HrmDbl=on
  Mux{1,3,5..11,14..24} (20 alike) : Mux  Inputs=N+1
  Mux{2,4,12..13} (4 alike) : DQN_Lib/Mux  N=N
  Mux52 : Mux  Inputs=2
  Mux57 : Mux  Inputs=2
  Mux58 : Mux  Inputs=2
  Product{1..3,5} (4 alike) : Product  Commented=on
  R_rec2 : Subsystem
  Rate Transition{1..5} (5 alike) : RateTransition  Integrity=off  OutPortSampleTimeMultiple=MultTs  OutPortSampleTime=Ts_Power
  Reshape{,1..7} (8 alike) : Reshape  OutputDimensionality=Customize  OutputDimensions=[N+1,6]
  Scope : Scope  NumInputPorts=2
  Scope11 : Scope  NumInputPorts=3
  Scope15 : Scope  Commented=on  NumInputPorts=2
  Scope8 : Scope  Commented=on  NumInputPorts=2
  Selector{,1..3} (4 alike) : Selector  InputPortWidth=3  IndexOptions=Index vector (dialog)  Indices=[1 2]  OutputSizes=1
  Selector4 : Selector  InputPortWidth=(N+1)*6  IndexOptions=Index vector (dialog)  Indices=(N+1)*5+1  OutputSizes=1
  Selector5 : Selector  InputPortWidth=(N+1)*6  IndexOptions=Index vector (dialog)  Indices=(N+1)*5+1  OutputSizes=1
  Subsystem1 : Subsystem  mask{Hi=4*HrmOrd, Ho=HrmOrd}
      mask prompts: Hi "Input harmonic order:"; Ho "Output harmonic order:"
  Subsystem2 : Subsystem  mask{Hi=4*HrmOrd, Ho=HrmOrd}
      mask prompts: Hi "Input harmonic order:"; Ho "Output harmonic order:"
  Subsystem3 : Subsystem  mask{Hi=4*HrmOrd, Ho=HrmOrd}
      mask prompts: Hi "Input harmonic order:"; Ho "Output harmonic order:"
  Subsystem4 : Subsystem  mask{Hi=4*HrmOrd, Ho=HrmOrd}
      mask prompts: Hi "Input harmonic order:"; Ho "Output harmonic order:"
  Subsystem5 : Subsystem  mask{Hi=4*HrmOrd, Ho=HrmOrd}
      mask prompts: Hi "Input harmonic order:"; Ho "Output harmonic order:"
  Subsystem6 : Subsystem  mask{Hi=4*HrmOrd, Ho=HrmOrd}
      mask prompts: Hi "Input harmonic order:"; Ho "Output harmonic order:"
  Subsystem7 : Subsystem  mask{Hi=4*HrmOrd, Ho=HrmOrd}
      mask prompts: Hi "Input harmonic order:"; Ho "Output harmonic order:"
  Subsystem8 : Subsystem  mask{Hi=4*HrmOrd, Ho=HrmOrd}
      mask prompts: Hi "Input harmonic order:"; Ho "Output harmonic order:"
  Subtract4 : Sum  Commented=on  Inputs=+-
  Subtract6 : Sum  Inputs=----
  Subtract8 : Sum  Commented=on  Inputs=+-
  Sum : Sum  Commented=on  Inputs=+
  Sum1 : Sum  Inputs=+-  InputSameDT=on  SaturateOnIntegerOverflow=on  OutDataTypeStr=Inherit: Same as first input
  Sum2 : Sum  Inputs=-+  InputSameDT=on  SaturateOnIntegerOverflow=on  OutDataTypeStr=Inherit: Same as first input
  Sum3 : Sum  Inputs=+-  InputSameDT=on  SaturateOnIntegerOverflow=on  OutDataTypeStr=Inherit: Same as first input
  Sum9 : Sum  Inputs=-+  InputSameDT=on  SaturateOnIntegerOverflow=on  OutDataTypeStr=Inherit: Same as first input
  Sum_DQN1 : DQN_Lib/Sum_DQN  HrmOrd=4*HrmOrd
  Sum_DQN2 : DQN_Lib/Sum_DQN  HrmOrd=4*HrmOrd
  Sum_DQN3 : DQN_Lib/Sum_DQN  HrmOrd=N
  sDQN2abc : DQN_Lib/sDQN2abc  HRM=4*HrmOrd
  sInt_DQN1 : DQN_Lib/sInt_DQN  HRM=HrmOrd  Ws=w  Ts=Ts_Power  HrmSeq=off
  sInt_DQN2 : DQN_Lib/sInt_DQN  HRM=HrmOrd  Ws=w  Ts=Ts_Power  HrmSeq=off
  sInt_DQN{4..7} (4 alike) : DQN_Lib/sInt_DQN  HRM=2*HrmOrd  Ws=w  Ts=Ts_Power  HrmSeq=off
  sInt_DQN_fdbk{1..4} (4 alike) : DQN_Lib/sInt_DQN_fdbk  HRM=4*HrmOrd  Ws=w  Ts=Ts_Power  HrmSeq=off  swFeed=on  R=R_arm  iL=1/(L_arm)
  sMult_DQN{1..3,8} (4 alike) : DQN_Lib/sMult_DQN  HRM=2*HrmOrd  HrmDbl=on  HrmSeq=off
  sMult_DQN{4..7} (4 alike) : DQN_Lib/sMult_DQN  HRM=HrmOrd  HrmDbl=on  HrmSeq=off
  Id_DQN_i : Outport  VectorParamsAs1DForOutWhenUnconnected=off
  Ig_DQN_i : Outport  Port=2  VectorParamsAs1DForOutWhenUnconnected=off
  Vg_DQN_i : Outport  Port=3  VectorParamsAs1DForOutWhenUnconnected=off
  Idc : Outport  Port=4  VectorParamsAs1DForOutWhenUnconnected=off
  Ig_DQN_r : Outport  Port=5  VectorParamsAs1DForOutWhenUnconnected=off
  Id_DQN_r : Outport  Port=6  VectorParamsAs1DForOutWhenUnconnected=off
  Vdc : Outport  Port=7  VectorParamsAs1DForOutWhenUnconnected=off
  wires:
  Gain15/1 -> Add4/2, Add5/2
  Discrete-Time Integrator5/1 -> Product2/1  "Vp_M"
  Add5/1 -> Product3/1
  Add4/1 -> Product1/1  "prod"
  Gain14/1 -> Discrete-Time Integrator5/1  "dVp_M"
  Product1/1 -> Gain14/1
  Discrete-Time Integrator4/1 -> Product5/1  "Vn_M"
  Gain13/1 -> Discrete-Time Integrator4/1  "dVn_M"
  Product3/1 -> Gain13/1
  From51/1 -> Product2/2, Product1/2
  From56/1 -> Product3/2, Product5/2
  From75/1 -> Scope8/2
  Constant/1 -> Subtract4/2
  Delay4/1 -> Gain54/1
  Gain55/1 -> Subtract8/2
  Subtract8/1 -> Delay4/1
  Gain53/1 -> Add36/1  "dVp_M"
  Gain52/1 -> Add36/2  "dVp_M"
  Add37/1 -> Scope8/1, Gain46/1  "prod"
  Subtract4/1 -> Subtract8/1
  Product2/1 -> Add35/1, Goto56/1
  Gain46/1 -> Scope15/1, Gain55/1, Gain15/1, Gain52/1, Gain53/1  "Igd"
  Product5/1 -> Add35/2, Goto57/1
  From72/1 -> Scope15/2
  Add36/1 -> Add37/1  "prod"
  Add35/1 -> Gain40/1
  Gain40/1 -> Add37/2  "Vce_i"
  From108/1 -> Add5/1, Add4/1
  Add10/1 -> sMult_DQN4/1  "prod"
  [Id_DQN_rc] -> Add16/1, Add10/1
  [mp_r_DQN] -> sMult_DQN1/2, sMult_DQN4/2
  Add16/1 -> sMult_DQN5/1
  [Ig_DQN_ic] -> Gain37/1
  [Id_DQN_ic] -> Add15/1, Add11/1
  sMult_DQN5/1 -> Gain31/1
  sInt_DQN5/1 -> sMult_DQN2/1  "Vn_M"
  [mp_i_DQN] -> sMult_DQN8/2, sMult_DQN7/2
  Add15/1 -> sMult_DQN7/1
  sInt_DQN6/1 -> sMult_DQN3/1  "Vp_M"
  sMult_DQN6/1 -> Gain35/1
  Gain36/1 -> Add16/2, Add10/2
  Gain35/1 -> sInt_DQN6/1  "dVp_M"
  [Ig_DQN_rc] -> Gain36/1
  Gain37/1 -> Add11/2, Add15/2
  Add11/1 -> sMult_DQN6/1  "prod"
  sMult_DQN7/1 -> Gain33/1
  sInt_DQN7/1 -> sMult_DQN8/1  "Vn_M"
  Gain33/1 -> sInt_DQN7/1  "dVn_M"
  Gain31/1 -> sInt_DQN5/1  "dVn_M"
  Gain34/1 -> sInt_DQN4/1  "dVp_M"
  [mn_r_DQN] -> sMult_DQN2/2, sMult_DQN5/2
  sMult_DQN4/1 -> Gain34/1
  [mn_i_DQN] -> sMult_DQN3/2, sMult_DQN6/2
  sInt_DQN4/1 -> sMult_DQN1/1  "Vp_M"
  Sum9/1 -> I->pu13/1
  Add17/1 -> Add20/1, Sum9/1  "dVp_M"
  [Vn_rc_DQN] -> Add17/2
  Add20/1 -> Sum_DQN1/1
  Add18/1 -> Add20/2, Sum3/2  "dVp_M"
  [Vp_ic_DQN] -> Add18/1
  [Vn_ic_DQN] -> Add18/2
  [Vp_rc_DQN] -> Add17/1
  Sum3/1 -> I->pu12/1
  [Vp_rc_DQN] -> Add9/1
  [Vn_rc_DQN] -> Add9/2
  Gain16/1 -> Add2/2  "dVp_M"
  Vg_DQN/1 -> Rate Transition4/1
  Add9/1 -> Subsystem1/1("{X_DQN}")
  Gain19/1 -> Add2/1  "dVp_M"
  Subtract6/1 -> Delay1/1
  Delay1/1 -> Gain20/1
  Gain20/1 -> sInt_DQN1/1, Gain19/1
  Add2/1 -> Subtract6/1  "prod"
  Gain11/1 -> Subtract6/2  "Vce_r"
  sInt_DQN1/1 -> [Ig_DQN_rc], R_rec2/1(In), Gain16/1  "Igd"
  sInt_DQN2/1 -> Add12/1
  Gain26/1 -> Add12/2  "dVp_M"
  Gain22/1 -> Delay3/1  "prod"
  Gain25/1 -> Gain29/1, [Ig_DQN_ic], Gain26/1  "Igd"
  Gain29/1 -> sInt_DQN2/1  "dVp_M"
  [Vp_ic_DQN] -> Add/1  "Vce_i"
  [Ig_DQN_rc] -> Gain1/1
  [Ig_DQN_ic] -> Ig_DQN_i/1  "Ig_DQN_i"
  [Id_DQN_ic] -> Id_DQN_i/1  "Id_DQN_i"
  [Vg_DQN_i] -> Vg_DQN_i/1  "Vg_DQN_i"
  [V_dc_c_DQN] -> Selector5/1  "Vdc"
  Gain1/1 -> Ig_DQN_r/1  "Ig_DQN_r"
  [Id_DQN_rc] -> Id_DQN_r/1  "Id_DQN_r"
  Gain38/1 -> Sum3/1, Subsystem2/1("{X_DQN}"), Sum9/2  "Vce_r"
  Gain41/1 -> Idc/1  "Vce_r"
  [Id_DQN_rc] -> Add1/2
  [Id_DQN_ic] -> Add1/1
  Selector4/1 -> Scope/1, Gain41/1  "Vdc"
  Sum_DQN1/1 -> Gain38/1
  Add1/1 -> Sum_DQN3/1
  Sum_DQN3/1 -> Scope/2, Selector4/1
  Add12/1 -> Add13/1  "Igd"
  R_rec2/1(Out) -> Subtract6/4
  Add13/1 -> Gain22/1  "prod"
  [Vn_ic_DQN] -> Add/2
  I->pu13/1 -> sInt_DQN_fdbk1/1
  I->pu12/1 -> sInt_DQN_fdbk2/1
  sInt_DQN_fdbk1/1 -> Delay7/1
  sInt_DQN_fdbk2/1 -> Delay8/1
  Delay3/1 -> Gain25/1, [Vg_DQN_i]
  Delay7/1 -> Subsystem4/1("{X_DQN}")
  Delay8/1 -> Subsystem5/1("{X_DQN}")
  Rate Transition4/1 -> Subtract6/3
  I->pu1/1 -> [mn_r_DQN]
  I->pu4/1 -> [mp_r_DQN]
  m_dq2_i/1 -> Rate Transition3/1
  m_dq1_i/1 -> Rate Transition5/1
  Mux18/1 -> Mux13/4
  Demux3/2 -> Mux9/3
  Mux20/1 -> Mux13/1
  Mux8/1 -> Mux2/2
  Mux5/1 -> Mux13/6
  Demux2/1 -> Mux7/2
  Constant3/1 -> Mux10/1
  Mux7/1 -> Mux2/1
  Constant4/1 -> Mux5/1
  Mux21/1 -> Mux13/5
  Demux1/2 -> Mux21/3
  Selector2/1 -> Demux1/1, Gain3/1
  Mux10/1 -> Mux2/6
  Mux14/1 -> Mux2/4
  Mux9/1 -> Mux2/5
  Demux/1 -> Mux20/2
  Demux/2 -> Mux18/2
  Gain3/1 -> Demux3/1
  Selector1/1 -> Demux2/1, Demux/1
  Demux2/2 -> Mux14/2
  Mux13/1 -> I->pu4/1
  m_dq1_r/1 -> Rate Transition1/1
  Demux3/1 -> Mux8/3
  m_dq2_r/1 -> Rate Transition2/1
  Mux3/1 -> Mux13/2
  Mux2/1 -> I->pu1/1
  Demux1/1 -> Mux3/3
  Rate Transition3/1 -> Selector3/1
  Mux11/1 -> Mux4/4
  Demux5/1 -> Mux15/3
  I->pu10/1 -> [mp_i_DQN]
  Mux23/1 -> Mux12/2
  Mux16/1 -> Mux4/5
  Constant6/1 -> Mux19/1
  Mux17/1 -> Mux12/1
  Mux19/1 -> Mux4/6
  Constant5/1 -> Mux1/1
  Selector3/1 -> Demux5/1, Gain6/1
  Demux4/2 -> Mux11/2
  Rate Transition5/1 -> Selector/1
  Gain6/1 -> Demux7/1
  Selector/1 -> Demux6/1, Demux4/1
  Demux7/1 -> Mux23/3
  I->pu9/1 -> [mn_i_DQN]
  Mux24/1 -> Mux12/5
  Mux6/1 -> Mux4/1
  Mux15/1 -> Mux4/2
  Demux7/2 -> Mux24/3
  Mux4/1 -> I->pu10/1
  Demux6/1 -> Mux17/2
  Mux22/1 -> Mux12/4
  Mux1/1 -> Mux12/6
  Mux12/1 -> I->pu9/1
  Demux5/2 -> Mux16/3
  Demux4/1 -> Mux6/2
  Demux6/2 -> Mux22/2
  Rate Transition2/1 -> Selector2/1
  Rate Transition1/1 -> Selector1/1
  sMult_DQN1/1 -> sDQN2abc/1, [Vp_rc_DQN]
  sMult_DQN2/1 -> [Vn_rc_DQN]
  sMult_DQN3/1 -> [Vp_ic_DQN]
  sMult_DQN8/1 -> [Vn_ic_DQN]
  Add/1 -> Subsystem3/1("{X_DQN}")
  Subsystem1/1("{Y_DQN}") -> Gain11/1
  Subsystem3/1("{Y_DQN}") -> Add13/2
  Subsystem4/1("{Y_DQN}") -> [Id_DQN_rc]
  Subsystem5/1("{Y_DQN}") -> [Id_DQN_ic]
  Selector5/1 -> Vdc/1  "Vdc"
  Subsystem2/1("{Y_DQN}") -> [V_dc_c_DQN]  "Vdc"
  [mp_i_DQN] -> Reshape2/1
  [mn_r_DQN] -> Reshape7/1
  Mult_DQNc_Mat4/1 -> Gain4/1
  Mult_DQNc_Mat3/1 -> Gain7/1
  Gain8/1 -> Add8/2, Add3/2
  [mn_i_DQN] -> Reshape4/1
  Mult_DQNc_Mat2/1 -> Gain5/1
  Int_DQNc_Mat2/1 -> Mult_DQNc_Mat6/1  "Vn_M"
  Add8/1 -> Mult_DQNc_Mat1/1
  Add7/1 -> Mult_DQNc_Mat4/1
  [mp_r_DQN] -> Reshape6/1
  Add6/1 -> Mult_DQNc_Mat3/1  "prod"
  Gain4/1 -> Int_DQNc_Mat4/1  "dVn_M"
  [Ig_DQN_ic] -> Reshape1/1
  Gain7/1 -> Int_DQNc_Mat3/1  "dVp_M"
  Int_DQNc_Mat4/1 -> Mult_DQNc_Mat8/1  "Vn_M"
  Int_DQNc_Mat3/1 -> Mult_DQNc_Mat7/1  "Vp_M"
  Gain5/1 -> Int_DQNc_Mat1/1  "dVp_M"
  Gain2/1 -> Int_DQNc_Mat2/1  "dVn_M"
  Gain9/1 -> Add6/2, Add7/2
  Mult_DQNc_Mat8/1 -> [Vn_ic_c]
  Add3/1 -> Mult_DQNc_Mat2/1  "prod"
  Mult_DQNc_Mat5/1 -> DQn->ABC9/1, [Vp_rc_c]
  Int_DQNc_Mat1/1 -> Mult_DQNc_Mat5/1  "Vp_M"
  Mult_DQNc_Mat6/1 -> [Vn_rc_c]
  [Id_DQN_rc] -> Reshape/1
  [Id_DQN_ic] -> Reshape3/1
  Mult_DQNc_Mat7/1 -> [Vp_ic_c]
  [Ig_DQN_rc] -> Reshape5/1
  Mult_DQNc_Mat1/1 -> Gain2/1
  MATLAB Function/1(Ydcpnz_c) -> Add8/1, Add3/1
  MATLAB Function1/1(Ydcpnz_c) -> Gain8/1
  MATLAB Function2/1(Ydcpnz_c) -> Add7/1, Add6/1
  MATLAB Function3/1(Ydcpnz_c) -> Gain9/1
  MATLAB Function4/1(Ydcpnz_c) -> Mult_DQNc_Mat5/2, Mult_DQNc_Mat2/2
  MATLAB Function5/1(Ydcpnz_c) -> Mult_DQNc_Mat6/2, Mult_DQNc_Mat1/2
  MATLAB Function6/1(Ydcpnz_c) -> Mult_DQNc_Mat7/2, Mult_DQNc_Mat3/2
  [theta0] -> DQn->ABC9/2, sDQN2abc/2
  Mux57/1 -> Scope11/1
  Mux52/1 -> Scope11/2
  DQn->ABC9/1 -> Demux35/1
  Demux34/1 -> Mux57/2
  sDQN2abc/1 -> Demux34/1
  Demux35/2 -> Mux52/1
  Demux34/3 -> Mux58/2
  Mux58/1 -> Scope11/3
  Demux35/3 -> Mux58/1
  Demux34/2 -> Mux52/2
  Demux35/1 -> Mux57/1
  MATLAB Function7/1(Ydcpnz_c) -> Mult_DQNc_Mat8/2, Mult_DQNc_Mat4/2
  Reshape/1 -> MATLAB Function/1(X_DQN)
  Reshape1/1 -> MATLAB Function3/1(X_DQN)
  Reshape2/1 -> MATLAB Function7/1(X_DQN)
  Reshape3/1 -> MATLAB Function2/1(X_DQN)
  Reshape4/1 -> MATLAB Function6/1(X_DQN)
  Reshape5/1 -> MATLAB Function1/1(X_DQN)
  Reshape6/1 -> MATLAB Function4/1(X_DQN)
  Reshape7/1 -> MATLAB Function5/1(X_DQN)
  [Vn_rc_c] -> Add14/2
  Delay5/1 -> Subsystem8/1("{X_DQN}")
  sInt_DQN_fdbk4/1 -> Delay5/1
  Add21/1 -> Sum_DQN2/1
  Delay2/1 -> Subsystem7/1("{X_DQN}")
  I->pu3/1 -> sInt_DQN_fdbk3/1
  Sum_DQN2/1 -> Gain10/1
  I->pu2/1 -> sInt_DQN_fdbk4/1
  sInt_DQN_fdbk3/1 -> Delay2/1
  Sum1/1 -> I->pu2/1
  [Vp_rc_c] -> Add14/1
  Sum2/1 -> I->pu3/1
  Subsystem6/1("{Y_DQN}") -> [V_dc_c_DQN]  "Vdc"
  [Vp_ic_c] -> Add19/1
  Subsystem8/1("{Y_DQN}") -> [Id_DQN_ic]
  [Vn_ic_c] -> Add19/2
  Subsystem7/1("{Y_DQN}") -> [Id_DQN_rc]
  Add14/1 -> Add21/1, Sum2/1  "dVp_M"
  Add19/1 -> Add21/2, Sum1/2  "dVp_M"
  Gain10/1 -> Sum1/1, Subsystem6/1("{X_DQN}"), Sum2/2  "Vce_r"
